simulink model "simulink_groundhook"  (R2020b)
settings: Solver=ode15s  StartTime=0  StopTime=10  MaxStep=0.001  RelTol=1e-3
values from neighbouring files (symbols this model uses):
  c2 = 100    [custom_main_groundhook.m]
  cG = cG_arr(idx)    [custom_main_groundhook.m]
  Gr = 2.56e-6    (= 2.56e-06)    [custom_main_groundhook.m]
  vcar = vcar_arra(idxcar)/3.6    [custom_main_groundhook.m]
  wcut = 2*pi*vcar/100    [custom_main_groundhook.m]
undefined symbols (not defined in the file or in its folder): SS
libraries: simulink x1, slctrlblks x1
settings Model: Creator=Slayer  LastModifiedBy=kevin
settings SFSimCC: CustomCodeUndefinedFunction=UseInterfaceOnly

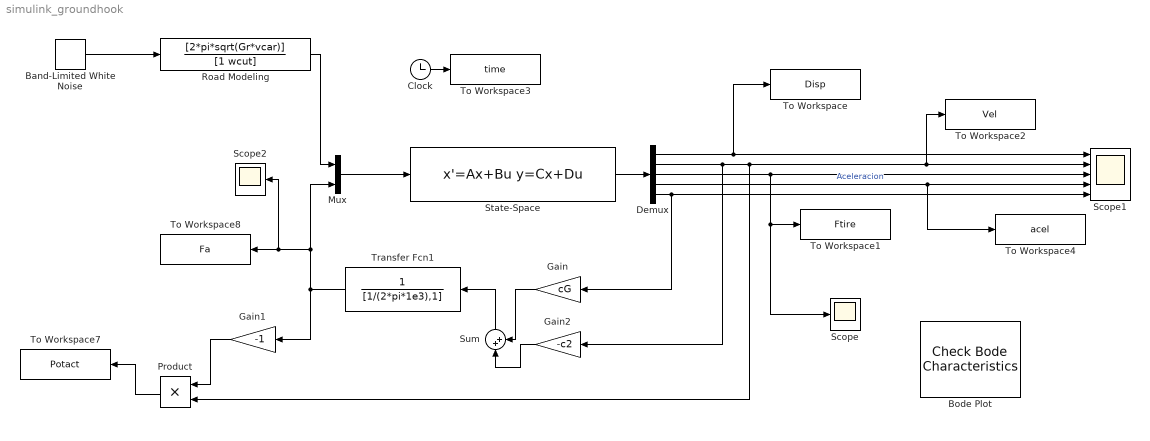
== system simulink_groundhook ==
  Band-Limited White Noise : simulink/Sources/Band-Limited White Noise  Cov=[0.5]  Ts=0.001  seed=[23341]
  Bode Plot : slctrlblks/Model Verification/Check Bode  Characteristics  InstantiateOnLoad=on  SaveOperatingPoints=off  LinearizationIOs={'/Road Modeling ', 1, 'in', 'off', '';'/Demux', 3, 'out', 'on', ''}  LinearizeAt=SnapshotTimes  SnapshotTimes=[0]  TriggerType=rising  SampleTime=auto  RateConversionMethod=zoh  PreWarpFreq=10  UseExactDelayModel=off  UseFullBlockNameLabels=off  UseBusSignalLabels=off  enabled=on  stopWhenAssertionFail=off  export=off  ViewDlgPos=[1250 115 510 390]  OpenViewOnLoad=off  LaunchViewOnOpen=on  FrequencyUnits=rad/s  MagnitudeUnits=dB  PhaseUnits=deg  TimeUnits=seconds  EnableUpperBound=off  UpperBoundFrequencies=[]  UpperBoundMagnitudes=[]  EnableLowerBound=off  LowerBoundFrequencies=[]  LowerBoundMagnitudes=[]
      settings: SaveToWorkspace=on  SaveName=ground
  Clock : Clock
  Demux : Demux  Outputs=5
  Gain : Gain  Gain=cG
  Gain1 : Gain  Gain=-1
  Gain2 : Gain  Gain=-c2
  Mux : Mux  Inputs=2
  Product : Product
  "Road Modeling " : TransferFcn  Numerator=[2*pi*sqrt(Gr*vcar)]  Denominator=[1 wcut]
  Scope : Scope
  Scope1 : Scope  NumInputPorts=5
  Scope2 : Scope
  State-Space : StateSpace  A=SS.A  B=SS.B  C=SS.C  D=SS.D  InitialCondition=0
  Sum : Sum  Inputs=|++
  To Workspace : ToWorkspace  VariableName=Disp  SampleTime=0.001
  To Workspace1 : ToWorkspace  VariableName=Ftire  SampleTime=0.001
  To Workspace2 : ToWorkspace  VariableName=Vel  SampleTime=0.001
  To Workspace3 : ToWorkspace  VariableName=time  SampleTime=0.001
  To Workspace4 : ToWorkspace  VariableName=acel  SampleTime=0.001
  To Workspace7 : ToWorkspace  VariableName=Potact  SampleTime=0.001
  To Workspace8 : ToWorkspace  VariableName=Fa  SampleTime=0.001
  Transfer Fcn1 : TransferFcn  Numerator=1  Denominator=[1/(2*pi*1e3),1]
  wires:
  Demux/2 -> Gain2/1, Product/2, To Workspace2/1, Scope1/2
  State-Space/1 -> Demux/1
  Demux/1 -> To Workspace/1, Scope1/1
  Demux/3 -> Scope1/3, Scope/1, To Workspace1/1
  Clock/1 -> To Workspace3/1
  Demux/4 -> To Workspace4/1, Scope1/4  "Aceleracion"
  Mux/1 -> State-Space/1
  Demux/5 -> Gain/1, Scope1/5
  Product/1 -> To Workspace7/1
  Band-Limited White Noise/1 -> "Road Modeling "/1
  "Road Modeling "/1 -> Mux/1
  Gain1/1 -> Product/1
  Gain/1 -> Sum/2
  Transfer Fcn1/1 -> Gain1/1, Scope2/1, To Workspace8/1, Mux/2
  Gain2/1 -> Sum/1
  Sum/1 -> Transfer Fcn1/1
